simulink model "nonlinear_model"  (R2020b)
settings: Solver=VariableStepAuto  StartTime=0.0  StopTime=10.0  RelTol=1e-3
settings Model: Creator=Zeyuan  LastModifiedBy=Zeyuan

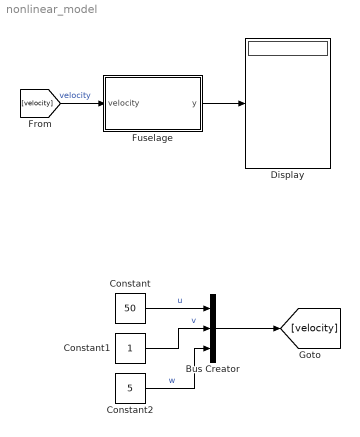
== system nonlinear_model ==
  Bus Creator : BusCreator  Inputs=3
  Constant : Constant  Value=50
  Constant1 : Constant
  Constant2 : Constant  Value=5
  Display : Display
  Fuselage : MATLAB Function  TreatAsAtomicUnit=on
  wires:
  [velocity] -> Fuselage/1(velocity)  "velocity"
  Bus Creator/1 -> [velocity]
  Constant/1 -> Bus Creator/1  "u"
  Constant1/1 -> Bus Creator/2  "v"
  Constant2/1 -> Bus Creator/3  "w"
  Fuselage/1(y) -> Display/1

== matlab function nonlinear_model/Fuselage ==
  data: velocity input; y output
function y = fcn(velocity)
%velocity: u,v,w
u_F = velocity(1);
v_F = velocity(2);
w_F = velocity(3);
rho = 1.2133;
R = 5.49;
A = pi*R^2;


if u_F == 0
    alpha_F = pi/2*sign(w_F);
elseif u_F > 0
    alpha_F = atan(w_F/u_F);
else
    alpha_F = pi + atan(w_F/u_F);
end

if u_F == 0
    beta_F = pi/2*sign(v_F);
elseif u_F > 0
    beta_F = atan(v_F/u_F);
else
    beta_F = pi + atan(v_F/u_F);
end
            

C_X0F = -0.0217;
C_X1F = 0.0602;
C_YF = -0.1721;
C_ZF = -0.0817;

X_F         = 1/2*rho*(u_F^2+v_F^2+w_F^2)*A*(C_X0F+C_X1F*alpha_F^2);
Y_F         = 1/2*rho*(u_F^2+v_F^2+w_F^2)*A*(C_YF*beta_F);
Z_F         = 1/2*rho*(u_F^2+v_F^2+w_F^2)*A*(C_ZF*alpha_F);

C_LF = 0;
C_MF = 0.0179;
C_NF = 0.0179;

L_F = 0;
M_F = 1/2*rho*(u_F^2+v_F^2+w_F^2)*A*2*R*(C_MF*alpha_F);
N_F = 1/2*rho*(u_F^2+v_F^2+w_F^2)*A*2*R*(C_NF*beta_F);
            

u = velocity(1);
v = velocity(2);
w = velocity(3);


y = [X_F;Y_F;Z_F;L_F;M_F;N_F];
